simulink model "ReplayFlight_ME_RTC_v9b"  (Simulink 7.5)
settings: Solver=FixedStepDiscrete  StartTime=0.0  StopTime=d_data(end,1)  FixedStep=apSampleTime  RelTol=1e-3
InitFcn:
  | replayFlight
values from neighbouring files (symbols this model uses):
  apSampleTime = 0.01    [demoz2SlugsV5.m]
  D = y    [BarOrthog.m]
  R0 = single(Euler2DCMdeg( PHI_IC, THETA_IC, PSI_IC ))    [demoz2SlugsV5.m]
undefined symbols (not defined in the file or in its folder): accBiasRateLimit, accelXCutTemp, axTGain1, axTGain2, axTMean1, axTMean2, barAdjust, baroCutoff, baroCutTemp, baroOffset, baroScale, barTGain1, barTGain2, barTMean1, barTMean2, baseHeight, baseTemp, cubeAccelGain, cubeGyroGain, gaind, GS_location, gyroBiasRateLimit, Init_onlyOnce, Init_Reset, ISA_rho0, lapseRate, lowRateSensorCutoff, magMeanTemp, magOffset, magScale, magTempK, mainSensorCutoff, maxDynPressure, param_acc, param_mag, pitAdjust, pitCutTemp, pitotOffset, pitotScale, pitTGain1, pitTGain2, pitTMean1, pitTMean2, polesd, powerOffset, powerScale, pressureSensorCutoff, T, tempOffset, tempScale, Vb_0, vzCutoff, xCutoff, yCutoff, zCutoff, zerosd
libraries: simulink x12, aerolibconvert2 x9, SLUGS_Library x6, aerolibutil x3, dspmtrx3 x3, dsPICdrivers x1
(part 2 of 4)

== system ReplayFlight_ME_RTC_v9b/Position and Attitude Filter/Geod2LTP1/ECEF2LTP (UEN) ==
  ECEF coordinates : Inport  OutDataType=sfix(16)  OutScaling=2^0
  "Long, Lat" : Inport  Port=2  OutDataType=sfix(16)  OutScaling=2^0
  Deg2R : Gain  Gain=pi/180  ParameterDataType=sfix(16)  ParameterScaling=2^0  OutDataType=sfix(16)  OutScaling=2^0  SaturateOnIntegerOverflow=on  OutDataTypeStr=Inherit: Same as input  ParamDataTypeStr=Inherit: Same as input
  Demux3 : Demux  Outputs=2
  From Body to Universal1 : Subsystem
  Product1 : Product  Multiplication=Matrix(*)  OutDataType=sfix(16)  OutScaling=2^0  SaturateOnIntegerOverflow=on  InputSameDT=on  OutDataTypeStr=Inherit: Same as first input
  Out : Outport  OutDataType=sfix(16)  OutScaling=2^0
  wires:
  "Long, Lat"/1 -> Deg2R/1
  Product1/1 -> Out/1
  Demux3/2 -> From Body to Universal1/2(lat)
  Demux3/1 -> From Body to Universal1/1(long)
  Deg2R/1 -> Demux3/1
  ECEF coordinates/1 -> Product1/2
  From Body to Universal1/1(DCM) -> Product1/1

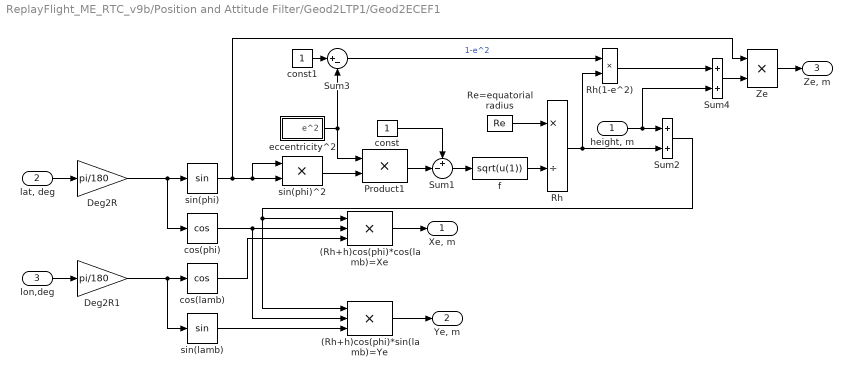
== system ReplayFlight_ME_RTC_v9b/Position and Attitude Filter/Geod2LTP1/Geod2ECEF1 ==
  "height, m" : Inport  OutDataType=sfix(16)  OutScaling=2^0
  "lat, deg" : Inport  Port=2  OutDataType=sfix(16)  OutScaling=2^0
  lon,deg : Inport  Port=3  OutDataType=sfix(16)  OutScaling=2^0
  (Rh+h)cos(phi)*cos(lamb)=Xe : Product  Inputs=3  OutDataTypeMode=single  OutDataType=sfix(16)  OutScaling=2^0  OutDataTypeStr=single  SaturateOnIntegerOverflow=on  InputSameDT=on
  (Rh+h)cos(phi)*sin(lamb)=Ye : Product  Inputs=3  OutDataTypeMode=single  OutDataType=sfix(16)  OutScaling=2^0  OutDataTypeStr=single  SaturateOnIntegerOverflow=on  InputSameDT=on
  Deg2R : Gain  Gain=pi/180  ParameterDataType=sfix(16)  ParameterScaling=2^0  OutDataTypeMode=Specify via dialog  OutDataType=float('single')  OutDataTypeStr=float('single')  SaturateOnIntegerOverflow=on  ParamDataTypeStr=Inherit: Same as input
  Deg2R1 : Gain  Gain=pi/180  ParameterDataType=sfix(16)  ParameterScaling=2^0  OutDataTypeMode=Specify via dialog  OutDataType=float('single')  OutDataTypeStr=float('single')  SaturateOnIntegerOverflow=on  ParamDataTypeStr=Inherit: Same as input
  Product1 : Product  OutDataType=sfix(16)  OutScaling=2^0  SaturateOnIntegerOverflow=on  InputSameDT=on  OutDataTypeStr=Inherit: Same as first input
  Re=equatorial radius : Constant  Value=Re  OutDataTypeMode=single  OutDataType=sfix(16)  OutScaling=2^0  OutDataTypeStr=single
  Rh : Product  Inputs=*/  OutDataTypeMode=single  OutDataType=sfix(16)  OutScaling=2^0  OutDataTypeStr=single  SaturateOnIntegerOverflow=on  InputSameDT=on
  Rh(1-e^2) : Product  OutDataTypeMode=single  OutDataType=sfix(16)  OutScaling=2^0  OutDataTypeStr=single  SaturateOnIntegerOverflow=on  InputSameDT=on
  Sum1 : Sum  Inputs=+-|  OutDataType=sfix(16)  OutScaling=2^0  SaturateOnIntegerOverflow=on  InputSameDT=on  OutDataTypeStr=Inherit: Same as first input
  Sum2 : Sum  OutDataType=sfix(16)  OutScaling=2^0  SaturateOnIntegerOverflow=on  InputSameDT=on  OutDataTypeStr=Inherit: Same as first input
      settings: AttributesFormatString=Rh+h
  Sum3 : Sum  Inputs=|+-  OutDataType=sfix(16)  OutScaling=2^0  SaturateOnIntegerOverflow=on  InputSameDT=on  OutDataTypeStr=Inherit: Same as first input
  Sum4 : Sum  OutDataTypeMode=single  OutDataType=sfix(16)  OutScaling=2^0  OutDataTypeStr=single  SaturateOnIntegerOverflow=on  InputSameDT=on
      settings: AttributesFormatString=(1-e^2)Rh+h
  Ze : Product  OutDataTypeMode=single  OutDataType=sfix(16)  OutScaling=2^0  OutDataTypeStr=single  SaturateOnIntegerOverflow=on  InputSameDT=on
  const : Constant  OutDataTypeMode=single  OutDataType=sfix(16)  OutScaling=2^0  OutDataTypeStr=single
  const1 : Constant  OutDataTypeMode=single  OutDataType=sfix(16)  OutScaling=2^0  OutDataTypeStr=single
  cos(lamb) : Trigonometry  Operator=cos
  cos(phi) : Trigonometry  Operator=cos
  eccentricity^2 : Subsystem
  f : Fcn  Expr=sqrt(u(1))
  sin(lamb) : Trigonometry
  sin(phi) : Trigonometry
  sin(phi)^2 : Product  OutDataType=sfix(16)  OutScaling=2^0  SaturateOnIntegerOverflow=on  InputSameDT=on  OutDataTypeStr=Inherit: Same as first input
  "Xe, m " : Outport  OutDataType=sfix(16)  OutScaling=2^0
  "Ye, m " : Outport  Port=2  OutDataType=sfix(16)  OutScaling=2^0
  "Ze, m " : Outport  Port=3  OutDataType=sfix(16)  OutScaling=2^0
  wires:
  "lat, deg"/1 -> Deg2R/1
  sin(phi)/1 -> sin(phi)^2/1, sin(phi)^2/2, Ze/1
  f/1 -> Rh/2
  Re=equatorial radius/1 -> Rh/1
  Rh/1 -> Sum2/2, Rh(1-e^2)/2
  Product1/1 -> Sum1/2
  Sum1/1 -> f/1
  const/1 -> Sum1/1
  "height, m"/1 -> Sum4/2, Sum2/1
  eccentricity^2/1(e^2) -> Product1/1, Sum3/2
  sin(phi)^2/1 -> Product1/2
  const1/1 -> Sum3/1
  Sum3/1 -> Rh(1-e^2)/1  "1-e^2"
  Rh(1-e^2)/1 -> Sum4/1
  Sum4/1 -> Ze/2
  lon,deg/1 -> Deg2R1/1
  cos(phi)/1 -> (Rh+h)cos(phi)*cos(lamb)=Xe/2, (Rh+h)cos(phi)*sin(lamb)=Ye/2
  cos(lamb)/1 -> (Rh+h)cos(phi)*cos(lamb)=Xe/3
  sin(lamb)/1 -> (Rh+h)cos(phi)*sin(lamb)=Ye/3
  Ze/1 -> "Ze, m "/1
  Deg2R/1 -> cos(phi)/1, sin(phi)/1
  Deg2R1/1 -> cos(lamb)/1, sin(lamb)/1
  Sum2/1 -> (Rh+h)cos(phi)*sin(lamb)=Ye/1, (Rh+h)cos(phi)*cos(lamb)=Xe/1
  (Rh+h)cos(phi)*cos(lamb)=Xe/1 -> "Xe, m "/1
  (Rh+h)cos(phi)*sin(lamb)=Ye/1 -> "Ye, m "/1

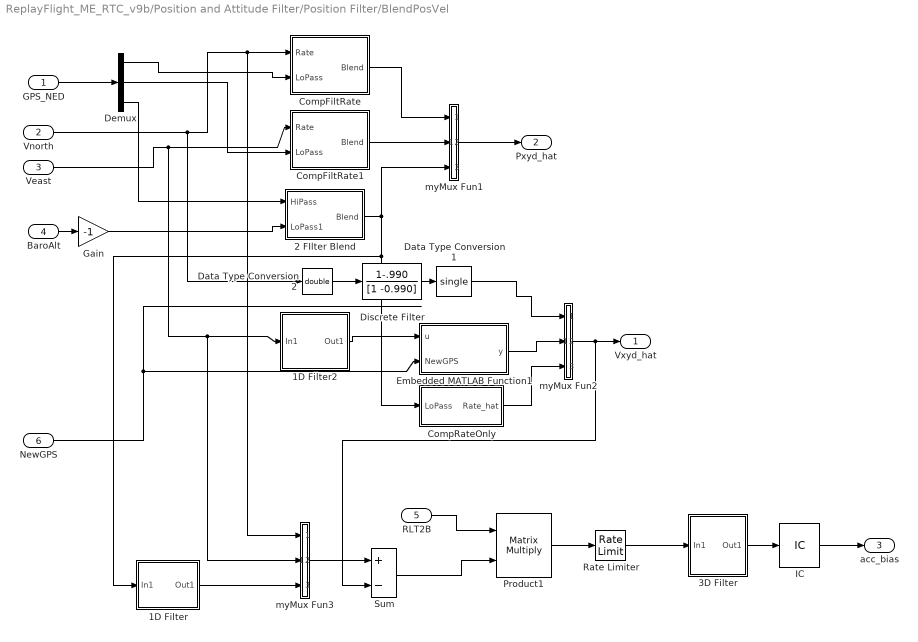
== system ReplayFlight_ME_RTC_v9b/Position and Attitude Filter/Position Filter/BlendPosVel ==
  GPS_NED : Inport  OutDataType=sfix(16)  OutScaling=2^0
  Vnorth : Inport  Port=2  OutDataType=sfix(16)  OutScaling=2^0
  Veast : Inport  Port=3  OutDataType=sfix(16)  OutScaling=2^0
  BaroAlt : Inport  Port=4  OutDataType=sfix(16)  OutScaling=2^0
  RLT2B : Inport  Port=5  OutDataType=sfix(16)  OutScaling=2^0
  NewGPS : Inport  Port=6  OutDataType=sfix(16)  OutScaling=2^0
  1D Filter : Subsystem  AncestorBlock=SLUGS_Library/Singnal Routing & Conditioning/3D Filter  RTWFcnName=TustinFilter3D  mask{zval=[0], pval=-50, kval=1, TSample=apSampleTime}
      mask prompts: zval "Zeros"; pval "Poles"; kval "Gains"; TSample "Sample Time"
      settings: RTWFcnNameOpts=User specified  RTWFileNameOpts=Use function name
      mask Display:
      | droots(zval,pval,kval)
      | port_label('input',1,'1D')
  1D Filter2 : Subsystem  AncestorBlock=SLUGS_Library/Singnal Routing & Conditioning/3D Filter  RTWFcnName=TustinFilter3D  mask{zval=[], pval=-5, kval=5, TSample=apSampleTime}
      mask prompts: zval "Zeros"; pval "Poles"; kval "Gains"; TSample "Sample Time"
      settings: RTWFcnNameOpts=User specified  RTWFileNameOpts=Use function name
      mask Display:
      | droots(zval,pval,kval)
      | port_label('input',1,'1D')
  2 FIlter Blend : Subsystem
  3D Filter : Subsystem  AncestorBlock=SLUGS_Library/Singnal Routing & Conditioning/3D Filter  RTWFcnName=TustinFilter3D  mask{zval=[], pval=[0], kval=1, TSample=0.01}
      mask prompts: zval "Zeros"; pval "Poles"; kval "Gains"; TSample "Sample Time"
      settings: RTWFcnNameOpts=User specified  RTWFileNameOpts=Use function name
      mask Display:
      | droots(zval,pval,kval)
      | port_label('input',1,'3D')
  CompFiltRate : Subsystem  mask{omega=xCutoff, T=apSampleTime}
      mask prompts: omega "Cutoff Freq (rad/sec)"; T "Sample Time"
  CompFiltRate1 : Subsystem  mask{omega=yCutoff, T=apSampleTime}
      mask prompts: omega "Cutoff Freq (rad/sec)"; T "Sample Time"
  CompRateOnly : Subsystem  mask{omega=vzCutoff, T=apSampleTime}
      mask prompts: omega "Cutoff Freq (rad/sec)"; T "Sample Time"
  Data Type Conversion1 : DataTypeConversion  OutDataTypeMode=single  OutDataType=sfix(16)  OutScaling=2^0  OutDataTypeStr=single
  Data Type Conversion2 : DataTypeConversion  OutDataTypeMode=double  OutDataType=sfix(16)  OutScaling=2^0  OutDataTypeStr=double
  Demux : Demux  Outputs=3
  Discrete Filter : DiscreteFilter  Numerator=1-.990  Denominator=[1 -0.990]
  Embedded MATLAB Function1 : Stateflow chart  TreatAsAtomicUnit=on
  Gain : Gain  Gain=-1  ParameterDataType=sfix(16)  ParameterScaling=2^0  OutDataType=sfix(16)  OutScaling=2^0
  IC : InitialCondition  Value=0
  Product1 : Product  Multiplication=Matrix(*)  OutDataType=sfix(16)  OutScaling=2^0  RndMeth=Zero
  Rate Limiter : RateLimiter  RisingSlewLimit=accBiasRateLimit  FallingSlewLimit=-accBiasRateLimit  SampleTimeMode=inherited
  Sum : Sum  Inputs=+-  OutDataTypeMode=single  OutDataType=sfix(16)  OutScaling=2^0  OutDataTypeStr=single
  myMux Fun1 : Stateflow chart  TreatAsAtomicUnit=on
  myMux Fun2 : Stateflow chart  TreatAsAtomicUnit=on
  myMux Fun3 : Stateflow chart  TreatAsAtomicUnit=on
  Vxyd_hat : Outport  OutDataType=sfix(16)  OutScaling=2^0
  Pxyd_hat : Outport  Port=2  OutDataType=sfix(16)  OutScaling=2^0
  acc_bias : Outport  Port=3  OutDataType=sfix(16)  OutScaling=2^0
  wires:
  GPS_NED/1 -> Demux/1
  Vnorth/1 -> myMux Fun3/1(u1), CompFiltRate/1(Rate), Data Type Conversion2/1
  Veast/1 -> CompFiltRate1/1(Rate), myMux Fun3/2(u2), 1D Filter2/1(In1)
  Demux/1 -> CompFiltRate/2(LoPass)
  Demux/2 -> CompFiltRate1/2(LoPass)
  BaroAlt/1 -> Gain/1
  Demux/3 -> 2 FIlter Blend/1(HiPass)
  CompFiltRate1/1(Blend) -> myMux Fun1/2(u2)
  CompFiltRate/1(Blend) -> myMux Fun1/1(u1)
  2 FIlter Blend/1(Blend) -> myMux Fun1/3(u3), CompRateOnly/1(LoPass), 1D Filter/1(In1)
  myMux Fun1/1(y) -> Pxyd_hat/1
  Gain/1 -> 2 FIlter Blend/2(LoPass1)
  NewGPS/1 -> Embedded MATLAB Function1/2(NewGPS)
  Embedded MATLAB Function1/1(y) -> myMux Fun2/2(u2)
  myMux Fun2/1(y) -> Vxyd_hat/1, Sum/2
  CompRateOnly/1(Rate_hat) -> myMux Fun2/3(u3)
  RLT2B/1 -> Product1/1
  Product1/1 -> Rate Limiter/1
  1D Filter/1(Out1) -> myMux Fun3/3(u3)
  myMux Fun3/1(y) -> Sum/1
  Sum/1 -> Product1/2
  3D Filter/1(Out1) -> IC/1
  Rate Limiter/1 -> 3D Filter/1(In1)
  1D Filter2/1(Out1) -> Embedded MATLAB Function1/1(u)
  Data Type Conversion1/1 -> myMux Fun2/1(u1)
  Data Type Conversion2/1 -> Discrete Filter/1
  Discrete Filter/1 -> Data Type Conversion1/1
  IC/1 -> acc_bias/1

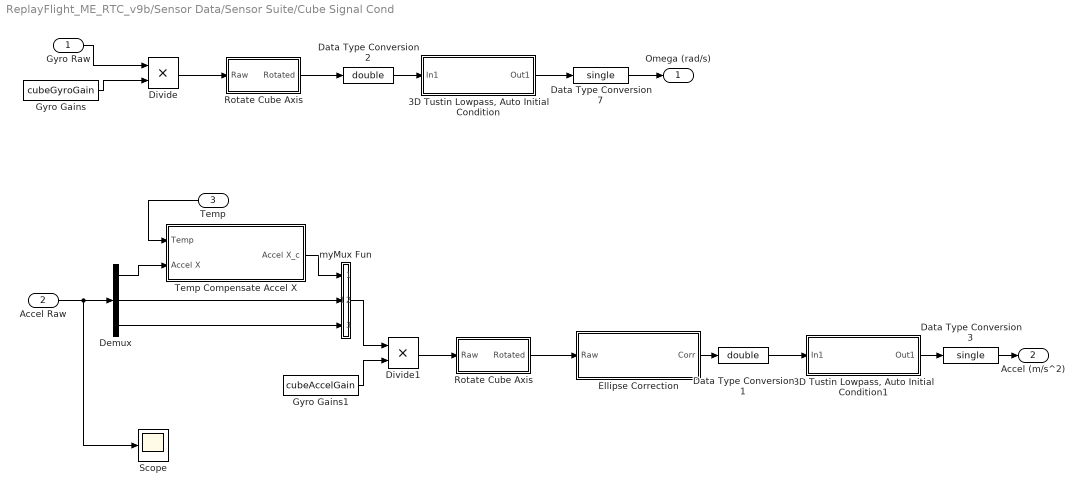
== system ReplayFlight_ME_RTC_v9b/Sensor Data/Sensor Suite/Cube Signal Cond ==
  Gyro Raw : Inport  OutDataType=sfix(16)  OutScaling=2^0
  Accel Raw : Inport  Port=2  OutDataType=sfix(16)  OutScaling=2^0
  Temp : Inport  Port=3  OutDataType=sfix(16)  OutScaling=2^0
  "3D Tustin Lowpass, Auto Initial Condition" : Subsystem  mask(Tustin1stOrderLowpassAutoInitialCondition){f=mainSensorCutoff, T=T}
      mask prompts: f "Lowpass Frequency"; T "Sample Time"
      mask help: Takes a 3db rolloff frequency (in Hz, NOT radians/s) and a sample time. Performs a symbolic Tustin conversion and implements in a discrete filter. The initial output of the filter is set by the first sample.
      mask Help: Enter the desired 3db rolloff frequency in Hz and the sample time. Initial conditions are sampled automatically.
      mask Display: fprintf('%.2f Hz lowpass (3D)',f)
  "3D Tustin Lowpass, Auto Initial Condition1" : Subsystem  mask(Tustin1stOrderLowpassAutoInitialCondition){f=mainSensorCutoff, T=T}
      mask prompts: f "Lowpass Frequency"; T "Sample Time"
      mask help: Takes a 3db rolloff frequency (in Hz, NOT radians/s) and a sample time. Performs a symbolic Tustin conversion and implements in a discrete filter. The initial output of the filter is set by the first sample.
      mask Help: Enter the desired 3db rolloff frequency in Hz and the sample time. Initial conditions are sampled automatically.
      mask Display: fprintf('%.2f Hz lowpass (3D)',f)
  Data Type Conversion1 : DataTypeConversion  OutDataTypeMode=double  OutDataType=sfix(16)  OutScaling=2^0  OutDataTypeStr=double
  Data Type Conversion2 : DataTypeConversion  OutDataTypeMode=double  OutDataType=sfix(16)  OutScaling=2^0  OutDataTypeStr=double
  Data Type Conversion3 : DataTypeConversion  OutDataTypeMode=single  OutDataType=sfix(16)  OutScaling=2^0  OutDataTypeStr=single
  Data Type Conversion7 : DataTypeConversion  OutDataTypeMode=single  OutDataType=sfix(16)  OutScaling=2^0  OutDataTypeStr=single
  Demux : Demux  Outputs=3
  Divide : Product  OutDataTypeMode=single  OutDataType=sfix(16)  OutScaling=2^-10  OutDataTypeStr=single
  Divide1 : Product  OutDataTypeMode=single  OutDataType=sfix(16)  OutScaling=2^-10  OutDataTypeStr=single
  Ellipse Correction : Subsystem  AncestorBlock=SLUGS_Library/Singnal Routing & Conditioning/Ellipse Correction  mask{param=param_acc}
      mask prompts: param "parameter (struct)"
      mask help: Applies the correction from the ellipse algorithm to the raw data being sent through the block. The block expects a 3x1 input vector, and will return a 3x1 output vector. The parameter constant should be a struct with param.xo .yo and .zo being the offsets, param.a .b and .c being the scale factors, and param.phi .rho and .lambda being the angle non-orthogonality (in degrees).
      mask Display:
      | text(0.2,0.85,'Ellipse Correction')
      | port_label('input',1,'RAW')
      | port_label('output',1,'CORR')
  Gyro Gains : Constant  Value=cubeGyroGain  OutDataTypeMode=single  OutDataType=sfix(16)  OutScaling=2^0  OutDataTypeStr=single
  Gyro Gains1 : Constant  Value=cubeAccelGain  OutDataTypeMode=single  OutDataType=sfix(16)  OutScaling=2^0  OutDataTypeStr=single
  Rotate Cube Axis : Subsystem
  "Rotate Cube Axis " : Subsystem
  Scope : Scope
      settings: YMin=-22.5  YMax=15  SaveName=ScopeData13
  Temp Compensate Accel X : Subsystem
  myMux Fun : Stateflow chart  TreatAsAtomicUnit=on
  Omega (rad/s) : Outport  OutDataType=sfix(16)  OutScaling=2^0
  Accel (m/s^2) : Outport  Port=2  OutDataType=sfix(16)  OutScaling=2^0
  wires:
  myMux Fun/1(y) -> Divide1/1
  Accel Raw/1 -> Demux/1, Scope/1
  Demux/1 -> Temp Compensate Accel X/2(Accel X)
  Temp Compensate Accel X/1(Accel X_c) -> myMux Fun/1(u1)
  Demux/3 -> myMux Fun/3(u3)
  Temp/1 -> Temp Compensate Accel X/1(Temp)
  Ellipse Correction/1(Corr) -> Data Type Conversion1/1
  Data Type Conversion3/1 -> Accel (m/s^2)/1
  "3D Tustin Lowpass, Auto Initial Condition1"/1(Out1) -> Data Type Conversion3/1
  Data Type Conversion1/1 -> "3D Tustin Lowpass, Auto Initial Condition1"/1(In1)
  Rotate Cube Axis/1(Rotated) -> Data Type Conversion2/1
  Data Type Conversion7/1 -> Omega (rad/s)/1
  "3D Tustin Lowpass, Auto Initial Condition"/1(Out1) -> Data Type Conversion7/1
  Data Type Conversion2/1 -> "3D Tustin Lowpass, Auto Initial Condition"/1(In1)
  Gyro Raw/1 -> Divide/1
  Gyro Gains1/1 -> Divide1/2
  "Rotate Cube Axis "/1(Rotated) -> Ellipse Correction/1(Raw)
  Divide1/1 -> "Rotate Cube Axis "/1(Raw)
  Divide/1 -> Rotate Cube Axis/1(Raw)
  Gyro Gains/1 -> Divide/2
  Demux/2 -> myMux Fun/2(u2)

== system ReplayFlight_ME_RTC_v9b/Sensor Data/Sensor Suite/If no HIL then Read all the Sensors ==
  Accel Raw : Subsystem
  Air Data : Subsystem
  Demux : Demux  Outputs=3
  Demux1 : Demux  Outputs=3
  Demux2 : Demux  Outputs=3
  Demux3 : Demux
  "GPS " : Subsystem
  Gyro Raw : Subsystem
  Mags : Subsystem
  Scope2 : Scope
      settings: YMin=315  YMax=375  SaveName=ScopeData12
  myMux Fun4 : Stateflow chart  TreatAsAtomicUnit=on
  Sensors : Outport  OutDataType=sfix(16)  OutScaling=2^0
  GPS : Outport  Port=2  OutDataType=sfix(16)  OutScaling=2^0
  wires:
  Mags/1(Mags) -> Demux1/1
  Demux1/3 -> myMux Fun4/9(u9)
  Demux1/2 -> myMux Fun4/8(u8)
  Demux1/1 -> myMux Fun4/7(u7)
  Demux/3 -> myMux Fun4/3(u3)
  Demux/2 -> myMux Fun4/2(u2)
  Demux/1 -> myMux Fun4/1(u1)
  myMux Fun4/1(y) -> Sensors/1
  Gyro Raw/1(Gyro) -> Demux/1
  Demux2/1 -> myMux Fun4/4(u4)
  Demux2/2 -> myMux Fun4/5(u5)
  Demux2/3 -> myMux Fun4/6(u6)
  Accel Raw/1(Accel) -> Demux2/1
  "GPS "/1(GPS) -> GPS/1
  Demux3/1 -> myMux Fun4/10(u10)
  Demux3/2 -> myMux Fun4/11(u11)
  Demux3/3 -> myMux Fun4/12(u12)
  Demux3/4 -> myMux Fun4/13(u13)
  Air Data/1(Air) -> Demux3/1, Scope2/1

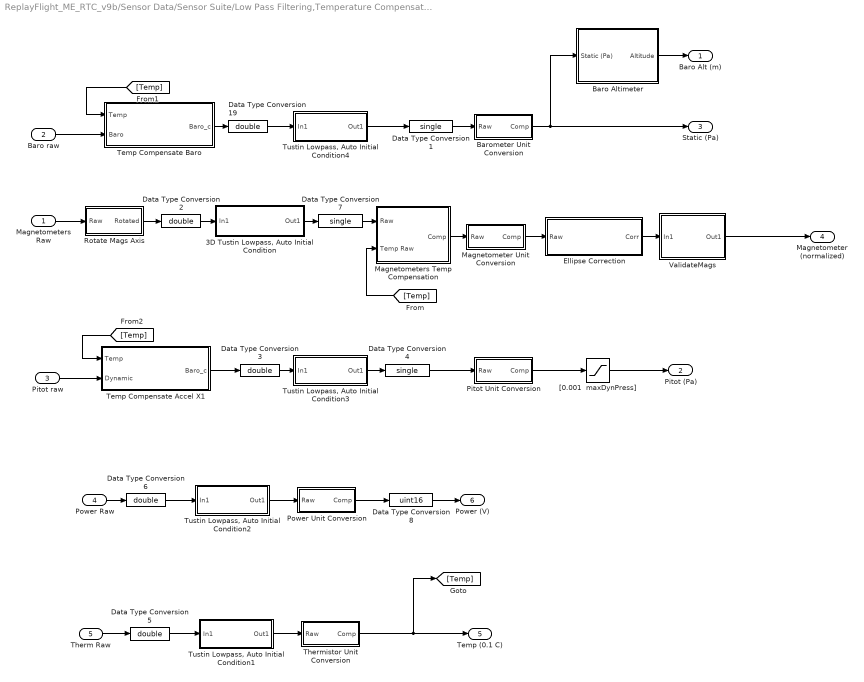
== system ReplayFlight_ME_RTC_v9b/Sensor Data/Sensor Suite/Low Pass Filtering,Temperature Compensation and Calibration ==
  Magnetometers Raw : Inport  OutDataType=sfix(16)  OutScaling=2^0
  Baro raw : Inport  Port=2  OutDataType=sfix(16)  OutScaling=2^0
  Pitot raw : Inport  Port=3  OutDataType=sfix(16)  OutScaling=2^0
  Power Raw : Inport  Port=4  OutDataType=sfix(16)  OutScaling=2^0
  Therm Raw : Inport  Port=5  OutDataType=sfix(16)  OutScaling=2^0
  "3D Tustin Lowpass, Auto Initial Condition" : Subsystem  mask(Tustin1stOrderLowpassAutoInitialCondition){f=mainSensorCutoff, T=T}
      mask prompts: f "Lowpass Frequency"; T "Sample Time"
      mask help: Takes a 3db rolloff frequency (in Hz, NOT radians/s) and a sample time. Performs a symbolic Tustin conversion and implements in a discrete filter. The initial output of the filter is set by the first sample.
      mask Help: Enter the desired 3db rolloff frequency in Hz and the sample time. Initial conditions are sampled automatically.
      mask Display: fprintf('%.2f Hz lowpass (3D)',f)
  Baro Altimeter : Subsystem
  Barometer Unit Conversion : Subsystem  mask{bias=baroOffset, gains=baroScale}
      mask prompts: bias "Initial Bias"; gains "Initial Gains"
      mask help: Convert Analog readings to units
  Data Type Conversion1 : DataTypeConversion  OutDataTypeMode=single  OutDataType=sfix(16)  OutScaling=2^0  OutDataTypeStr=single
  Data Type Conversion{2..3,5..6,19} (5 alike) : DataTypeConversion  OutDataTypeMode=double  OutDataType=sfix(16)  OutScaling=2^0  OutDataTypeStr=double
  Data Type Conversion4 : DataTypeConversion  OutDataTypeMode=single  OutDataType=sfix(16)  OutScaling=2^0  OutDataTypeStr=single
  Data Type Conversion7 : DataTypeConversion  OutDataTypeMode=single  OutDataType=sfix(16)  OutScaling=2^0  OutDataTypeStr=single
  Data Type Conversion8 : DataTypeConversion  OutDataTypeMode=uint16  OutDataType=sfix(16)  OutScaling=2^0  OutDataTypeStr=uint16
  Ellipse Correction : Subsystem  AncestorBlock=SLUGS_Library/Singnal Routing & Conditioning/Ellipse Correction  mask{param=param_mag}
      mask prompts: param "parameter (struct)"
      mask help: Applies the correction from the ellipse algorithm to the raw data being sent through the block. The block expects a 3x1 input vector, and will return a 3x1 output vector. The parameter constant should be a struct with param.xo .yo and .zo being the offsets, param.a .b and .c being the scale factors, and param.phi .rho and .lambda being the angle non-orthogonality (in degrees).
      mask Display:
      | text(0.2,0.85,'Ellipse Correction')
      | port_label('input',1,'RAW')
      | port_label('output',1,'CORR')
  Magnetometer Unit Conversion : Subsystem  mask{bias=magOffset, gains=magScale}
      mask prompts: bias "Initial Bias"; gains "Initial Gains"
      mask help: Convert Analog readings to units
  Magnetometers Temp Compensation : Subsystem  mask{alpha=magTempK, tempMean=magMeanTemp}
      mask prompts: alpha "Tempearature Coeficient (K_t)"; tempMean "Calibration Temperature Mean (T_avg)"
      mask help:
      | This block implements a temperature compensation. It implmements the following equation:
      |
      | M_tc = M_raw - K_t(T - T_avg)
  Pitot Unit Conversion : Subsystem  mask{bias=pitotOffset, gains=pitotScale}
      mask prompts: bias "Initial Bias"; gains "Initial Gains"
      mask help: Convert Analog readings to units
  Power Unit Conversion : Subsystem  mask{bias=powerOffset, gains=powerScale}
      mask prompts: bias "Initial Bias"; gains "Initial Gains"
      mask help: Convert Analog readings to units
  Rotate Mags Axis : Subsystem
  Temp Compensate Accel X1 : Subsystem
  Temp Compensate Baro : Subsystem
  Thermistor Unit Conversion : Subsystem  mask{bias=tempOffset, gains=tempScale}
      mask prompts: bias "Initial Bias"; gains "Initial Gains"
      mask help: Convert Analog readings to units
  "Tustin Lowpass, Auto Initial Condition1" : Subsystem  mask(Tustin1stOrderLowpassAutoInitialCondition){f=lowRateSensorCutoff, T=T}
      mask prompts: f "Lowpass Frequency"; T "Sample Time"
      mask help: Takes a 3db rolloff frequency (in Hz, NOT radians/s) and a sample time. Performs a symbolic Tustin conversion and implements in a discrete filter. The initial output of the filter is set by the first sample.
      mask Help: Enter the desired 3db rolloff frequency in Hz and the sample time. Initial conditions are sampled automatically.
      mask Display: fprintf('%.2f Hz lowpass',f)
  "Tustin Lowpass, Auto Initial Condition2" : Subsystem  mask(Tustin1stOrderLowpassAutoInitialCondition){f=lowRateSensorCutoff, T=T}
      mask prompts: f "Lowpass Frequency"; T "Sample Time"
      mask help: Takes a 3db rolloff frequency (in Hz, NOT radians/s) and a sample time. Performs a symbolic Tustin conversion and implements in a discrete filter. The initial output of the filter is set by the first sample.
      mask Help: Enter the desired 3db rolloff frequency in Hz and the sample time. Initial conditions are sampled automatically.
      mask Display: fprintf('%.2f Hz lowpass',f)
  "Tustin Lowpass, Auto Initial Condition3" : Subsystem  mask(Tustin1stOrderLowpassAutoInitialCondition){f=pressureSensorCutoff, T=T}
      mask prompts: f "Lowpass Frequency"; T "Sample Time"
      mask help: Takes a 3db rolloff frequency (in Hz, NOT radians/s) and a sample time. Performs a symbolic Tustin conversion and implements in a discrete filter. The initial output of the filter is set by the first sample.
      mask Help: Enter the desired 3db rolloff frequency in Hz and the sample time. Initial conditions are sampled automatically.
      mask Display: fprintf('%.2f Hz lowpass',f)
  "Tustin Lowpass, Auto Initial Condition4" : Subsystem  mask(Tustin1stOrderLowpassAutoInitialCondition){f=pressureSensorCutoff, T=T}
      mask prompts: f "Lowpass Frequency"; T "Sample Time"
      mask help: Takes a 3db rolloff frequency (in Hz, NOT radians/s) and a sample time. Performs a symbolic Tustin conversion and implements in a discrete filter. The initial output of the filter is set by the first sample.
      mask Help: Enter the desired 3db rolloff frequency in Hz and the sample time. Initial conditions are sampled automatically.
      mask Display: fprintf('%.2f Hz lowpass',f)
  ValidateMags : Subsystem
  "[0.001  maxDynPress]" : Saturate  UpperLimit=maxDynPressure  LowerLimit=0.001
  Baro Alt (m) : Outport  OutDataType=sfix(16)  OutScaling=2^0
  Pitot (Pa) : Outport  Port=2  OutDataType=sfix(16)  OutScaling=2^0
  Static (Pa) : Outport  Port=3  OutDataType=sfix(16)  OutScaling=2^0
  Magnetometer (normalized) : Outport  Port=4  OutDataType=sfix(16)  OutScaling=2^0
  Temp (0.1 C) : Outport  Port=5  OutDataType=sfix(16)  OutScaling=2^0
  Power (V) : Outport  Port=6  OutDataType=sfix(16)  OutScaling=2^0
  wires:
  Temp Compensate Accel X1/1(Baro_c) -> Data Type Conversion3/1
  Pitot raw/1 -> Temp Compensate Accel X1/2(Dynamic)
  [Temp] -> Temp Compensate Accel X1/1(Temp)
  Baro raw/1 -> Temp Compensate Baro/2(Baro)
  [Temp] -> Temp Compensate Baro/1(Temp)
  Temp Compensate Baro/1(Baro_c) -> Data Type Conversion19/1
  ValidateMags/1(Out1) -> Magnetometer (normalized)/1
  Ellipse Correction/1(Corr) -> ValidateMags/1(In1)
  Rotate Mags Axis/1(Rotated) -> Data Type Conversion2/1
  Magnetometer Unit Conversion/1(Comp) -> Ellipse Correction/1(Raw)
  Power Unit Conversion/1(Comp) -> Data Type Conversion8/1
  Pitot Unit Conversion/1(Comp) -> "[0.001  maxDynPress]"/1
  Baro Altimeter/1(Altitude) -> Baro Alt (m)/1
  Data Type Conversion8/1 -> Power (V)/1
  "Tustin Lowpass, Auto Initial Condition2"/1(Out1) -> Power Unit Conversion/1(Raw)
  Power Raw/1 -> Data Type Conversion6/1
  Data Type Conversion6/1 -> "Tustin Lowpass, Auto Initial Condition2"/1(In1)
  Thermistor Unit Conversion/1(Comp) -> [Temp], Temp (0.1 C)/1
  Data Type Conversion1/1 -> Barometer Unit Conversion/1(Raw)
  "Tustin Lowpass, Auto Initial Condition4"/1(Out1) -> Data Type Conversion1/1
  [Temp] -> Magnetometers Temp Compensation/2(Temp Raw)
  Magnetometers Temp Compensation/1(Comp) -> Magnetometer Unit Conversion/1(Raw)
  Data Type Conversion7/1 -> Magnetometers Temp Compensation/1(Raw)
  Data Type Conversion4/1 -> Pitot Unit Conversion/1(Raw)
  Magnetometers Raw/1 -> Rotate Mags Axis/1(Raw)
  Barometer Unit Conversion/1(Comp) -> Baro Altimeter/1(Static (Pa)), Static (Pa)/1
  Therm Raw/1 -> Data Type Conversion5/1
  Data Type Conversion5/1 -> "Tustin Lowpass, Auto Initial Condition1"/1(In1)
  "Tustin Lowpass, Auto Initial Condition3"/1(Out1) -> Data Type Conversion4/1
  Data Type Conversion3/1 -> "Tustin Lowpass, Auto Initial Condition3"/1(In1)
  Data Type Conversion19/1 -> "Tustin Lowpass, Auto Initial Condition4"/1(In1)
  "[0.001  maxDynPress]"/1 -> Pitot (Pa)/1
  "Tustin Lowpass, Auto Initial Condition1"/1(Out1) -> Thermistor Unit Conversion/1(Raw)
  "3D Tustin Lowpass, Auto Initial Condition"/1(Out1) -> Data Type Conversion7/1
  Data Type Conversion2/1 -> "3D Tustin Lowpass, Auto Initial Condition"/1(In1)

== system ReplayFlight_ME_RTC_v9b/Position and Attitude Filter/Attitude Complimentary Filter COG/3D Filter/Filter1 ==
  In1 : Inport  OutDataType=sfix(16)  OutScaling=2^0
  Discrete Zero-Pole : DiscreteZeroPole  Zeros=zerosd  Poles=polesd  Gain=gaind  SampleTime=SampleTime
  Out1 : Outport  OutDataType=sfix(16)  OutScaling=2^0
  wires:
  In1/1 -> Discrete Zero-Pole/1
  Discrete Zero-Pole/1 -> Out1/1

== system ReplayFlight_ME_RTC_v9b/Position and Attitude Filter/Attitude Complimentary Filter COG/3D Filter/Filter2 ==
  In1 : Inport  OutDataType=sfix(16)  OutScaling=2^0
  Discrete Zero-Pole : DiscreteZeroPole  Zeros=zerosd  Poles=polesd  Gain=gaind  SampleTime=SampleTime
  Out1 : Outport  OutDataType=sfix(16)  OutScaling=2^0
  wires:
  Discrete Zero-Pole/1 -> Out1/1
  In1/1 -> Discrete Zero-Pole/1

== system ReplayFlight_ME_RTC_v9b/Position and Attitude Filter/Attitude Complimentary Filter COG/3D Filter/Filter3 ==
  In1 : Inport  OutDataType=sfix(16)  OutScaling=2^0
  Discrete Zero-Pole : DiscreteZeroPole  Zeros=zerosd  Poles=polesd  Gain=gaind  SampleTime=SampleTime
  Out1 : Outport  OutDataType=sfix(16)  OutScaling=2^0
  wires:
  In1/1 -> Discrete Zero-Pole/1
  Discrete Zero-Pole/1 -> Out1/1

== system ReplayFlight_ME_RTC_v9b/Position and Attitude Filter/Attitude Complimentary Filter COG/3D Filter2/Filter1 ==
  In1 : Inport  OutDataType=sfix(16)  OutScaling=2^0
  Discrete Zero-Pole : DiscreteZeroPole  Zeros=zerosd  Poles=polesd  Gain=gaind  SampleTime=SampleTime
  Out1 : Outport  OutDataType=sfix(16)  OutScaling=2^0
  wires:
  In1/1 -> Discrete Zero-Pole/1
  Discrete Zero-Pole/1 -> Out1/1

== system ReplayFlight_ME_RTC_v9b/Position and Attitude Filter/Attitude Complimentary Filter COG/3D Filter2/Filter2 ==
  In1 : Inport  OutDataType=sfix(16)  OutScaling=2^0
  Discrete Zero-Pole : DiscreteZeroPole  Zeros=zerosd  Poles=polesd  Gain=gaind  SampleTime=SampleTime
  Out1 : Outport  OutDataType=sfix(16)  OutScaling=2^0
  wires:
  Discrete Zero-Pole/1 -> Out1/1
  In1/1 -> Discrete Zero-Pole/1

== system ReplayFlight_ME_RTC_v9b/Position and Attitude Filter/Attitude Complimentary Filter COG/3D Filter2/Filter3 ==
  In1 : Inport  OutDataType=sfix(16)  OutScaling=2^0
  Discrete Zero-Pole : DiscreteZeroPole  Zeros=zerosd  Poles=polesd  Gain=gaind  SampleTime=SampleTime
  Out1 : Outport  OutDataType=sfix(16)  OutScaling=2^0
  wires:
  In1/1 -> Discrete Zero-Pole/1
  Discrete Zero-Pole/1 -> Out1/1

== system ReplayFlight_ME_RTC_v9b/Position and Attitude Filter/Attitude Complimentary Filter COG/Direction Cosine Matrix to Euler Angles/cos(phi)cos(theta) ==
  DCM : Inport  OutDataType=sfix(16)  OutScaling=2^0
  Demux : Demux  Outputs=9
  Terminator{,1..7} (8 alike) : Terminator
  cos(phi)cos(theta) : Outport  OutDataType=sfix(16)  OutScaling=2^0
  wires:
  Demux/4 -> Terminator/1
  Demux/3 -> Terminator1/1
  Demux/5 -> Terminator4/1
  Demux/2 -> Terminator3/1
  Demux/1 -> Terminator2/1
  DCM/1 -> Demux/1
  Demux/8 -> Terminator7/1
  Demux/6 -> Terminator5/1
  Demux/7 -> Terminator6/1
  Demux/9 -> cos(phi)cos(theta)/1

== system ReplayFlight_ME_RTC_v9b/Position and Attitude Filter/Attitude Complimentary Filter COG/Direction Cosine Matrix to Euler Angles/cos(psi)cos(theta) ==
  DCM : Inport  OutDataType=sfix(16)  OutScaling=2^0
  Demux : Demux  Outputs=9
  Terminator{,1..7} (8 alike) : Terminator
  cos(psi)cos(theta) : Outport  OutDataType=sfix(16)  OutScaling=2^0
  wires:
  Demux/9 -> Terminator2/1
  Demux/7 -> Terminator6/1
  Demux/6 -> Terminator5/1
  Demux/8 -> Terminator7/1
  DCM/1 -> Demux/1
  Demux/1 -> cos(psi)cos(theta)/1
  Demux/2 -> Terminator3/1
  Demux/5 -> Terminator4/1
  Demux/3 -> Terminator1/1
  Demux/4 -> Terminator/1

== system ReplayFlight_ME_RTC_v9b/Position and Attitude Filter/Attitude Complimentary Filter COG/Direction Cosine Matrix to Euler Angles/sin(phi)cos(theta) ==
  DCM : Inport  OutDataType=sfix(16)  OutScaling=2^0
  Demux : Demux  Outputs=9
  Terminator{,1..7} (8 alike) : Terminator
  sin(phi)cos(theta) : Outport  OutDataType=sfix(16)  OutScaling=2^0
  wires:
  Demux/9 -> Terminator7/1
  Demux/7 -> Terminator6/1
  Demux/6 -> Terminator5/1
  Demux/8 -> sin(phi)cos(theta)/1
  DCM/1 -> Demux/1
  Demux/1 -> Terminator2/1
  Demux/2 -> Terminator3/1
  Demux/5 -> Terminator4/1
  Demux/3 -> Terminator1/1
  Demux/4 -> Terminator/1

== system ReplayFlight_ME_RTC_v9b/Position and Attitude Filter/Attitude Complimentary Filter COG/Direction Cosine Matrix to Euler Angles/sin(psi)cos(theta) ==
  DCM : Inport  OutDataType=sfix(16)  OutScaling=2^0
  Demux : Demux  Outputs=9
  Terminator{,1..7} (8 alike) : Terminator
  sin(psi)cos(theta) : Outport  OutDataType=sfix(16)  OutScaling=2^0
  wires:
  Demux/4 -> sin(psi)cos(theta)/1
  Demux/3 -> Terminator1/1
  Demux/5 -> Terminator4/1
  Demux/2 -> Terminator3/1
  Demux/1 -> Terminator2/1
  DCM/1 -> Demux/1
  Demux/8 -> Terminator/1
  Demux/6 -> Terminator5/1
  Demux/7 -> Terminator6/1
  Demux/9 -> Terminator7/1

== system ReplayFlight_ME_RTC_v9b/Position and Attitude Filter/Attitude Complimentary Filter COG/Direction Cosine Matrix to Euler Angles/sin(theta) ==
  DCM : Inport  OutDataType=sfix(16)  OutScaling=2^0
  Demux : Demux  Outputs=9
  Gain2 : Gain  Gain=-1  ParameterDataType=sfix(16)  ParameterScaling=2^0  OutDataType=sfix(16)  OutScaling=2^0  SaturateOnIntegerOverflow=on  OutDataTypeStr=Inherit: Same as input  ParamDataTypeStr=Inherit: Same as input
  Terminator{,1..5,7..8} (8 alike) : Terminator
  sin(theta) : Outport  OutDataType=sfix(16)  OutScaling=2^0
  wires:
  Gain2/1 -> sin(theta)/1
  Demux/4 -> Terminator/1
  Demux/3 -> Terminator1/1
  Demux/5 -> Terminator4/1
  Demux/2 -> Terminator3/1
  Demux/1 -> Terminator2/1
  DCM/1 -> Demux/1
  Demux/8 -> Terminator8/1
  Demux/6 -> Terminator5/1
  Demux/7 -> Gain2/1
  Demux/9 -> Terminator7/1

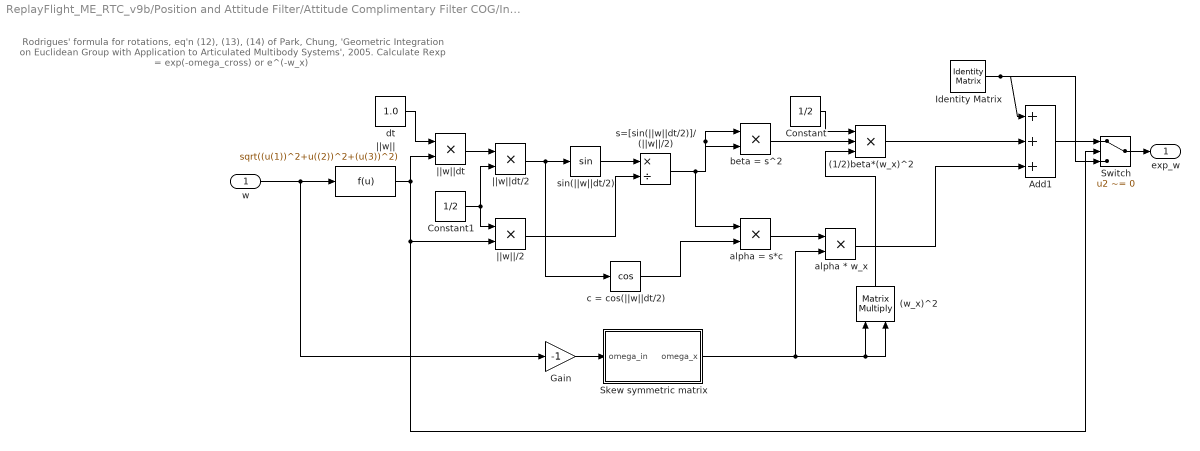
== system ReplayFlight_ME_RTC_v9b/Position and Attitude Filter/Attitude Complimentary Filter COG/IntegrateGyrosMatrixExp/Rexp, Rodrigues formula ==
  note: Rodrigues' formula for rotations, eq'n (12), (13), (14) of
      | Park, Chung, 'Geometric Integration on Euclidean
      | Group with Application to Articulated Multibody Systems', 2005.
      | Calculate Rexp = exp(-omega_cross) or e^(-w_x)
  w : Inport
  (1/2)beta*(w_x)^2 : Product  Inputs=3  OutDataTypeMode=double  OutDataType=fixdt(1, 16)  OutScaling=2^0  OutDataTypeStr=double  RndMeth=Zero
  (w_x)^2 : Product  Multiplication=Matrix(*)  OutDataTypeMode=double  OutDataType=fixdt(1, 16)  OutScaling=2^0  OutDataTypeStr=double  RndMeth=Zero
  Add1 : Sum  Inputs=+++  AccumDataTypeStr=double  OutDataType=sfix(16)  OutScaling=2^-10
  Constant : Constant  Value=1/2  OutDataTypeMode=double  OutDataType=fixdt(1, 16)  OutScaling=2^0  OutDataTypeStr=double
  Constant1 : Constant  Value=1/2  OutDataTypeMode=double  OutDataType=fixdt(1, 16)  OutScaling=2^0  OutDataTypeStr=double
  Gain : Gain  Gain=-1  ParameterDataType=fixdt(1, 16)  ParameterScaling=2^0  OutDataTypeMode=double  OutDataType=fixdt(1, 16)  OutScaling=2^0  OutDataTypeStr=double
  Identity Matrix : dspmtrx3/Identity Matrix  Inherit=off  N=3  Ts=inf  dataType=double  isSigned=on  wordLen=16  udDataType=sfix(16)  fracBitsMode=Best precision  numFracBits=15
  Skew symmetric matrix : Subsystem
  Switch : Switch  Criteria=u2 ~= 0  OutDataType=fixdt(1, 16)  OutScaling=2^0
  alpha * w_x : Product  OutDataTypeMode=double  OutDataType=fixdt(1, 16)  OutScaling=2^0  OutDataTypeStr=double  RndMeth=Zero
  alpha = s*c : Product  OutDataTypeMode=double  OutDataType=fixdt(1, 16)  OutScaling=2^0  OutDataTypeStr=double  RndMeth=Zero
  beta = s^2 : Product  OutDataTypeMode=double  OutDataType=fixdt(1, 16)  OutScaling=2^0  OutDataTypeStr=double  RndMeth=Zero
  c = cos(||w||dt/2) : Trigonometry  Operator=cos  OutputSignalType=real
  dt : Constant  Value=1.0  OutDataTypeMode=double  OutDataType=fixdt(1, 16)  OutScaling=2^0  OutDataTypeStr=double
  s=[sin(||w||dt/2)]/ (||w||/2) : Product  Inputs=*/  OutDataType=fixdt(1, 16)  OutScaling=2^-10
  sin(||w||dt/2) : Trigonometry  OutputSignalType=real
  ||w|| : Fcn  Expr=sqrt((u(1))^2+u((2))^2+(u(3))^2)
  ||w||/2 : Product  OutDataType=fixdt(1, 16)  OutScaling=2^0  RndMeth=Zero
  "||w||dt " : Product  OutDataType=fixdt(1, 16)  OutScaling=2^0  RndMeth=Zero
  ||w||dt/2 : Product  OutDataType=fixdt(1, 16)  OutScaling=2^0  RndMeth=Zero
  exp_w : Outport
  wires:
  Skew symmetric matrix/1(omega_x) -> (w_x)^2/1, (w_x)^2/2, alpha * w_x/2
  w/1 -> Gain/1, ||w||/1
  Identity Matrix/1 -> Add1/1, Switch/3
  Gain/1 -> Skew symmetric matrix/1(omega_in)
  c = cos(||w||dt/2)/1 -> alpha = s*c/2
  alpha = s*c/1 -> alpha * w_x/1
  alpha * w_x/1 -> Add1/3
  (1/2)beta*(w_x)^2/1 -> Add1/2
  Constant/1 -> (1/2)beta*(w_x)^2/1
  beta = s^2/1 -> (1/2)beta*(w_x)^2/2
  (w_x)^2/1 -> (1/2)beta*(w_x)^2/3
  s=[sin(||w||dt/2)]/ (||w||/2)/1 -> beta = s^2/1, beta = s^2/2, alpha = s*c/1
  dt/1 -> "||w||dt "/1
  ||w||/1 -> "||w||dt "/2, ||w||/2/2, Switch/2
  "||w||dt "/1 -> ||w||dt/2/1
  Constant1/1 -> ||w||dt/2/2, ||w||/2/1
  ||w||dt/2/1 -> sin(||w||dt/2)/1, c = cos(||w||dt/2)/1
  sin(||w||dt/2)/1 -> s=[sin(||w||dt/2)]/ (||w||/2)/1
  ||w||/2/1 -> s=[sin(||w||dt/2)]/ (||w||/2)/2
  Add1/1 -> Switch/1
  Switch/1 -> exp_w/1

== system ReplayFlight_ME_RTC_v9b/Position and Attitude Filter/Compute GS Location/Geod2ECEF1/eccentricity^2 ==
  " " : Product  OutDataTypeMode=single  OutDataType=sfix(16)  OutScaling=2^0  OutDataTypeStr=single  SaturateOnIntegerOverflow=on  InputSameDT=on
  Re=equatorial radius1 : Constant  Value=Re  OutDataTypeMode=single  OutDataType=sfix(16)  OutScaling=2^0  OutDataTypeStr=single
  Rp=polar radius : Constant  Value=Rp  OutDataTypeMode=single  OutDataType=sfix(16)  OutScaling=2^0  OutDataTypeStr=single
  Sum5 : Sum  Inputs=|+-  OutDataType=sfix(16)  OutScaling=2^0  SaturateOnIntegerOverflow=on  InputSameDT=on  OutDataTypeStr=Inherit: Same as first input
  const2 : Constant  OutDataTypeMode=single  OutDataType=sfix(16)  OutScaling=2^0  OutDataTypeStr=single
  e^1 : Product  Inputs=*/  OutDataTypeMode=single  OutDataType=sfix(16)  OutScaling=2^0  OutDataTypeStr=single  SaturateOnIntegerOverflow=on  InputSameDT=on
  e^2 : Outport  OutDataType=sfix(16)  OutScaling=2^0
  wires:
  Re=equatorial radius1/1 -> e^1/2
  Rp=polar radius/1 -> e^1/1
  const2/1 -> Sum5/1
  e^1/1 -> " "/2, " "/1
  " "/1 -> Sum5/2
  Sum5/1 -> e^2/1

== system ReplayFlight_ME_RTC_v9b/Position and Attitude Filter/Geod2LTP1/ECEF2LTP (UEN)/From Body to Universal1 ==
  long : Inport  OutDataType=sfix(16)  OutScaling=2^0
  lat : Inport  Port=2  OutDataType=sfix(16)  OutScaling=2^0
  Mux : Mux  Inputs=2
  Reshape 9x1->3x1 : S-Function  FunctionName=sreshape  Parameters=OutputDimensionality, OutputDimensions  EnableBusSupport=off  mask(Reshape){OutputDimensionality=Customize, OutputDimensions=[3,3]}
      mask prompts: OutputDimensionality "Output dimensionality:"; OutputDimensions "Output dimensions:"
      mask help:
      | Change the dimensions of a vector or matrix input signal. Output
      |  - a one-dimensional array (vector),
      |  - a column vector (Mx1 matrix),
      |  - a row vector (1xN matrix), or
      |  - a matrix or vector with specified dimensions, e.g., [M, N] or [W].
      mask init:
      | s = reshapemask(gcb,'init');
      mask StyleString: popup(1-D array|Column vector|Row vector|Customize),edit
      mask CallbackString: reshapemask(gcb,'cbDimensionality')|
      mask Display: disp('Reshape')
  Rotation Matrix from Long//Lat : Subsystem
      mask Type: Vector Transformation
      mask Description: Vector Transformation
      mask Display: disp('axis')
  DCM : Outport  OutDataType=sfix(16)  OutScaling=2^0
  wires:
  lat/1 -> Mux/2
  long/1 -> Mux/1
  Mux/1 -> Rotation Matrix from Long//Lat/1(long lat)
  Rotation Matrix from Long//Lat/1(DCM) -> Reshape 9x1->3x1/1
  Reshape 9x1->3x1/1 -> DCM/1

== system ReplayFlight_ME_RTC_v9b/Position and Attitude Filter/Geod2LTP1/Geod2ECEF1/eccentricity^2 ==
  " " : Product  OutDataTypeMode=single  OutDataType=sfix(16)  OutScaling=2^0  OutDataTypeStr=single  SaturateOnIntegerOverflow=on  InputSameDT=on
  Re=equatorial radius1 : Constant  Value=Re  OutDataTypeMode=single  OutDataType=sfix(16)  OutScaling=2^0  OutDataTypeStr=single
  Rp=polar radius : Constant  Value=Rp  OutDataTypeMode=single  OutDataType=sfix(16)  OutScaling=2^0  OutDataTypeStr=single
  Sum5 : Sum  Inputs=|+-  OutDataType=sfix(16)  OutScaling=2^0  SaturateOnIntegerOverflow=on  InputSameDT=on  OutDataTypeStr=Inherit: Same as first input
  const2 : Constant  OutDataTypeMode=single  OutDataType=sfix(16)  OutScaling=2^0  OutDataTypeStr=single
  e^1 : Product  Inputs=*/  OutDataTypeMode=single  OutDataType=sfix(16)  OutScaling=2^0  OutDataTypeStr=single  SaturateOnIntegerOverflow=on  InputSameDT=on
  e^2 : Outport  OutDataType=sfix(16)  OutScaling=2^0
  wires:
  Re=equatorial radius1/1 -> e^1/2
  Rp=polar radius/1 -> e^1/1
  const2/1 -> Sum5/1
  e^1/1 -> " "/2, " "/1
  " "/1 -> Sum5/2
  Sum5/1 -> e^2/1

== system ReplayFlight_ME_RTC_v9b/Position and Attitude Filter/Position Filter/BlendPosVel/1D Filter ==
  In1 : Inport  OutDataType=sfix(16)  OutScaling=2^0
  Data Type Conversion1 : DataTypeConversion  OutDataTypeMode=single  OutDataType=sfix(16)  OutScaling=2^0  OutDataTypeStr=single
  Data Type Conversion2 : DataTypeConversion  OutDataTypeMode=double  OutDataType=sfix(16)  OutScaling=2^0  OutDataTypeStr=double
  Filter2 : Subsystem  mask(DiscretizedZeroPole){Zeros=zval, Poles=pval, Gain=kval, AbsTol=auto, SampleTime=TSample, method=tustin, Wc=1}
      mask prompts: Zeros "Zeros (enter in s-main:)"; Poles "Poles (enter in s-domain:)"; Gain "Gain (enter in s-domain:)"; AbsTol "Absolute tolerance:"; SampleTime "Sample time:"; Wc "Critical Frequency (Hz):"
      mask help: Continuous mask uses c2d to transform parameters onto the Discrete Zero-Pole block inside.
      mask init: same as ReplayFlight_ME_RTC_v9b/Position and Attitude Filter/Attitude Complimentary Filter COG/3D Filter/Filter1
      mask StyleString: edit,edit,edit,edit,edit,popup(zoh|foh|tustin|prewarp|matched),edit
      mask CallbackString: |||||hidecrit|
      mask Display:
      | droots(zeross,poless,gainss)
      | text( 0.5, 1.0, method, 'verticalAlignment','top')
  Out1 : Outport  OutDataType=sfix(16)  OutScaling=2^0
  wires:
  Data Type Conversion1/1 -> Out1/1
  Data Type Conversion2/1 -> Filter2/1(In1)
  In1/1 -> Data Type Conversion2/1
  Filter2/1(Out1) -> Data Type Conversion1/1

== system ReplayFlight_ME_RTC_v9b/Position and Attitude Filter/Position Filter/BlendPosVel/1D Filter2 ==
  In1 : Inport  OutDataType=sfix(16)  OutScaling=2^0
  Data Type Conversion1 : DataTypeConversion  OutDataTypeMode=single  OutDataType=sfix(16)  OutScaling=2^0  OutDataTypeStr=single
  Data Type Conversion2 : DataTypeConversion  OutDataTypeMode=double  OutDataType=sfix(16)  OutScaling=2^0  OutDataTypeStr=double
  Filter2 : Subsystem  mask(DiscretizedZeroPole){Zeros=zval, Poles=pval, Gain=kval, AbsTol=auto, SampleTime=TSample, method=tustin, Wc=1}
      mask prompts: Zeros "Zeros (enter in s-main:)"; Poles "Poles (enter in s-domain:)"; Gain "Gain (enter in s-domain:)"; AbsTol "Absolute tolerance:"; SampleTime "Sample time:"; Wc "Critical Frequency (Hz):"
      mask help: Continuous mask uses c2d to transform parameters onto the Discrete Zero-Pole block inside.
      mask init: same as ReplayFlight_ME_RTC_v9b/Position and Attitude Filter/Attitude Complimentary Filter COG/3D Filter/Filter1
      mask StyleString: edit,edit,edit,edit,edit,popup(zoh|foh|tustin|prewarp|matched),edit
      mask CallbackString: |||||hidecrit|
      mask Display:
      | droots(zeross,poless,gainss)
      | text( 0.5, 1.0, method, 'verticalAlignment','top')
  Out1 : Outport  OutDataType=sfix(16)  OutScaling=2^0
  wires:
  Data Type Conversion1/1 -> Out1/1
  Data Type Conversion2/1 -> Filter2/1(In1)
  In1/1 -> Data Type Conversion2/1
  Filter2/1(Out1) -> Data Type Conversion1/1

== system ReplayFlight_ME_RTC_v9b/Position and Attitude Filter/Position Filter/BlendPosVel/2 FIlter Blend ==
  HiPass : Inport  OutDataType=sfix(16)  OutScaling=2^0
  LoPass1 : Inport  Port=2  OutDataType=sfix(16)  OutScaling=2^0
  1D Filter : Subsystem  AncestorBlock=SLUGS_Library/Singnal Routing & Conditioning/3D Filter  RTWFcnName=TustinFilter3D  mask{zval=[], pval=-zCutoff, kval=zCutoff, TSample=apSampleTime}
      mask prompts: zval "Zeros"; pval "Poles"; kval "Gains"; TSample "Sample Time"
      settings: RTWFcnNameOpts=User specified  RTWFileNameOpts=Use function name
      mask Display:
      | droots(zval,pval,kval)
      | port_label('input',1,'1D')
  1D Filter1 : Subsystem  AncestorBlock=SLUGS_Library/Singnal Routing & Conditioning/3D Filter  RTWFcnName=TustinFilter3D  mask{zval=[], pval=-baroCutoff, kval=baroCutoff, TSample=apSampleTime}
      mask prompts: zval "Zeros"; pval "Poles"; kval "Gains"; TSample "Sample Time"
      settings: RTWFcnNameOpts=User specified  RTWFileNameOpts=Use function name
      mask Display:
      | droots(zval,pval,kval)
      | port_label('input',1,'1D')
  Sum : Sum  OutDataTypeMode=single  OutDataType=sfix(16)  OutScaling=2^0  OutDataTypeStr=single
  Blend : Outport  OutDataType=sfix(16)  OutScaling=2^0
  wires:
  HiPass/1 -> 1D Filter/1(In1)
  LoPass1/1 -> 1D Filter1/1(In1)
  1D Filter/1(Out1) -> Sum/1
  1D Filter1/1(Out1) -> Sum/2
  Sum/1 -> Blend/1

== system ReplayFlight_ME_RTC_v9b/Position and Attitude Filter/Position Filter/BlendPosVel/3D Filter ==
  In1 : Inport  OutDataType=sfix(16)  OutScaling=2^0
  Data Type Conversion1 : DataTypeConversion  OutDataTypeMode=single  OutDataType=sfix(16)  OutScaling=2^0  OutDataTypeStr=single
  Data Type Conversion2 : DataTypeConversion  OutDataTypeMode=double  OutDataType=sfix(16)  OutScaling=2^0  OutDataTypeStr=double
  Demux : Demux  Outputs=3
  Filter1 : Subsystem  mask(DiscretizedZeroPole){Zeros=zval, Poles=pval, Gain=kval, AbsTol=auto, SampleTime=TSample, method=tustin, Wc=1}
      mask prompts: Zeros "Zeros (enter in s-main:)"; Poles "Poles (enter in s-domain:)"; Gain "Gain (enter in s-domain:)"; AbsTol "Absolute tolerance:"; SampleTime "Sample time:"; Wc "Critical Frequency (Hz):"
      mask help: Continuous mask uses c2d to transform parameters onto the Discrete Zero-Pole block inside.
      mask init: same as ReplayFlight_ME_RTC_v9b/Position and Attitude Filter/Attitude Complimentary Filter COG/3D Filter/Filter1
      mask StyleString: edit,edit,edit,edit,edit,popup(zoh|foh|tustin|prewarp|matched),edit
      mask CallbackString: |||||hidecrit|
      mask Display:
      | droots(zeross,poless,gainss)
      | text( 0.5, 1.0, method, 'verticalAlignment','top')
  Filter2 : Subsystem  mask(DiscretizedZeroPole){Zeros=zval, Poles=pval, Gain=kval, AbsTol=auto, SampleTime=TSample, method=tustin, Wc=1}
      mask prompts: Zeros "Zeros (enter in s-main:)"; Poles "Poles (enter in s-domain:)"; Gain "Gain (enter in s-domain:)"; AbsTol "Absolute tolerance:"; SampleTime "Sample time:"; Wc "Critical Frequency (Hz):"
      mask help: Continuous mask uses c2d to transform parameters onto the Discrete Zero-Pole block inside.
      mask init: same as ReplayFlight_ME_RTC_v9b/Position and Attitude Filter/Attitude Complimentary Filter COG/3D Filter/Filter1
      mask StyleString: edit,edit,edit,edit,edit,popup(zoh|foh|tustin|prewarp|matched),edit
      mask CallbackString: |||||hidecrit|
      mask Display:
      | droots(zeross,poless,gainss)
      | text( 0.5, 1.0, method, 'verticalAlignment','top')
  Filter3 : Subsystem  mask(DiscretizedZeroPole){Zeros=zval, Poles=pval, Gain=kval, AbsTol=auto, SampleTime=TSample, method=tustin, Wc=1}
      mask prompts: Zeros "Zeros (enter in s-main:)"; Poles "Poles (enter in s-domain:)"; Gain "Gain (enter in s-domain:)"; AbsTol "Absolute tolerance:"; SampleTime "Sample time:"; Wc "Critical Frequency (Hz):"
      mask help: Continuous mask uses c2d to transform parameters onto the Discrete Zero-Pole block inside.
      mask init: same as ReplayFlight_ME_RTC_v9b/Position and Attitude Filter/Attitude Complimentary Filter COG/3D Filter/Filter1
      mask StyleString: edit,edit,edit,edit,edit,popup(zoh|foh|tustin|prewarp|matched),edit
      mask CallbackString: |||||hidecrit|
      mask Display:
      | droots(zeross,poless,gainss)
      | text( 0.5, 1.0, method, 'verticalAlignment','top')
  myMux Fun1 : Stateflow chart  TreatAsAtomicUnit=on
  Out1 : Outport  OutDataType=sfix(16)  OutScaling=2^0
  wires:
  Data Type Conversion1/1 -> Out1/1
  Data Type Conversion2/1 -> Demux/1
  Demux/1 -> Filter1/1(In1)
  Demux/2 -> Filter2/1(In1)
  Demux/3 -> Filter3/1(In1)
  Filter1/1(Out1) -> myMux Fun1/1(u1)
  Filter2/1(Out1) -> myMux Fun1/2(u2)
  Filter3/1(Out1) -> myMux Fun1/3(u3)
  In1/1 -> Data Type Conversion2/1
  myMux Fun1/1(y) -> Data Type Conversion1/1

== system ReplayFlight_ME_RTC_v9b/Position and Attitude Filter/Position Filter/BlendPosVel/CompFiltRate ==
  Rate : Inport  OutDataType=sfix(16)  OutScaling=2^0
  LoPass : Inport  Port=2  OutDataType=sfix(16)  OutScaling=2^0
  1D Filter1 : Subsystem  AncestorBlock=SLUGS_Library/Singnal Routing & Conditioning/3D Filter  RTWFcnName=TustinFilter3D  mask{zval=[], pval=[0], kval=1, TSample=T}
      mask prompts: zval "Zeros"; pval "Poles"; kval "Gains"; TSample "Sample Time"
      settings: RTWFcnNameOpts=User specified  RTWFileNameOpts=Use function name
      mask Display:
      | droots(zval,pval,kval)
      | port_label('input',1,'1D')
  Gain : Gain  Gain=omega  ParameterDataType=sfix(16)  ParameterScaling=2^0  OutDataType=sfix(16)  OutScaling=2^0
  Sum : Sum  Inputs=++|  OutDataType=sfix(16)  OutScaling=2^0
  Sum1 : Sum  Inputs=|+-  OutDataType=sfix(16)  OutScaling=2^0
  Unit Delay : UnitDelay  SampleTime=T
  Blend : Outport  OutDataType=sfix(16)  OutScaling=2^0
  wires:
  1D Filter1/1(Out1) -> Blend/1, Unit Delay/1
  Sum/1 -> 1D Filter1/1(In1)
  Rate/1 -> Sum/1
  Gain/1 -> Sum/2
  Sum1/1 -> Gain/1
  LoPass/1 -> Sum1/1
  Unit Delay/1 -> Sum1/2

== system ReplayFlight_ME_RTC_v9b/Position and Attitude Filter/Position Filter/BlendPosVel/CompFiltRate1 ==
  Rate : Inport  OutDataType=sfix(16)  OutScaling=2^0
  LoPass : Inport  Port=2  OutDataType=sfix(16)  OutScaling=2^0
  1D Filter1 : Subsystem  AncestorBlock=SLUGS_Library/Singnal Routing & Conditioning/3D Filter  RTWFcnName=TustinFilter3D  mask{zval=[], pval=[0], kval=1, TSample=T}
      mask prompts: zval "Zeros"; pval "Poles"; kval "Gains"; TSample "Sample Time"
      settings: RTWFcnNameOpts=User specified  RTWFileNameOpts=Use function name
      mask Display:
      | droots(zval,pval,kval)
      | port_label('input',1,'1D')
  Gain : Gain  Gain=omega  ParameterDataType=sfix(16)  ParameterScaling=2^0  OutDataType=sfix(16)  OutScaling=2^0
  Sum : Sum  Inputs=++|  OutDataType=sfix(16)  OutScaling=2^0
  Sum1 : Sum  Inputs=|+-  OutDataType=sfix(16)  OutScaling=2^0
  Unit Delay : UnitDelay  SampleTime=T
  Blend : Outport  OutDataType=sfix(16)  OutScaling=2^0
  wires:
  1D Filter1/1(Out1) -> Blend/1, Unit Delay/1
  Sum/1 -> 1D Filter1/1(In1)
  Rate/1 -> Sum/1
  Gain/1 -> Sum/2
  Sum1/1 -> Gain/1
  LoPass/1 -> Sum1/1
  Unit Delay/1 -> Sum1/2

== system ReplayFlight_ME_RTC_v9b/Position and Attitude Filter/Position Filter/BlendPosVel/CompRateOnly ==
  LoPass : Inport  OutDataType=sfix(16)  OutScaling=2^0
  1D Filter1 : Subsystem  AncestorBlock=SLUGS_Library/Singnal Routing & Conditioning/3D Filter  RTWFcnName=TustinFilter3D  mask{zval=[], pval=[0], kval=1, TSample=T}
      mask prompts: zval "Zeros"; pval "Poles"; kval "Gains"; TSample "Sample Time"
      settings: RTWFcnNameOpts=User specified  RTWFileNameOpts=Use function name
      mask Display:
      | droots(zval,pval,kval)
      | port_label('input',1,'1D')
  Gain : Gain  Gain=omega  ParameterDataType=sfix(16)  ParameterScaling=2^0  OutDataType=sfix(16)  OutScaling=2^0
  Sum1 : Sum  Inputs=|+-  OutDataType=sfix(16)  OutScaling=2^0
  Unit Delay : UnitDelay  SampleTime=T
  Rate_hat : Outport  OutDataType=sfix(16)  OutScaling=2^0
  wires:
  1D Filter1/1(Out1) -> Unit Delay/1
  Gain/1 -> 1D Filter1/1(In1), Rate_hat/1
  Sum1/1 -> Gain/1
  LoPass/1 -> Sum1/1
  Unit Delay/1 -> Sum1/2
